simulink model "s32k344_mcb_sensorless_s32ct"  (R2024b)
settings: Solver=FixedStepAuto  StartTime=0.0  StopTime=20  RelTol=1e-3  EnableMultiTasking=on
PreLoadFcn:
  | % NXP_MBDT_S32K3 callback: DO NOT REMOVE
  | mbd_s32k3.common.nxp.model_callbacks.preLoadFcn();
  | 
  | s32k344Data;
  | mcbSensorlessData;
PostLoadFcn:
  | % NXP_MBDT_S32K3 callback: DO NOT REMOVE
  | mbd_s32k3.common.nxp.model_callbacks.postLoadFcn();
InitFcn:
  | % NXP_MBDT_S32K3 callback: DO NOT REMOVE
  | mbd_s32k3.common.nxp.model_callbacks.initFcn();
values from neighbouring files (symbols this model uses):
  PWM_DutyScale = 32768    [s32k344Data.m]
  PWM_Period = 8000    [s32k344Data.m]
  Ts_motor = T_pwm    (= 5e-05)    [s32k344Data.m]
  Ts_SerialIn = 0.1    [s32k344Data.m]
  Ts_SerialOut = 0.01    [s32k344Data.m]
  Ts_SysControl = 0.1    [mcbSensorlessData.m]
undefined symbols (not defined in the file or in its folder): inverter, LogicOutputId, pmsm, Value
libraries: mbd_s32k3_io_library x14, mbd_s32k3_cdd_library x4, simulink x4, mbd_s32k3_isr_library x1, mbd_s32k3_utility_library x1
(part 3 of 3)

== system s32k344_mcb_sensorless_s32ct/Control/HW INT/CodeGeneration/ADC_INT/ADC_IRQHandler/Fault Detection ==
  VDC : Inport
  Constant : Constant  Value=pmsm.V_max/inverter.MaxADCCnt  OutDataTypeStr=single  SampleTime=-1
  Data Type Conversion : DataTypeConversion  OutDataTypeStr=single  SaturateOnIntegerOverflow=off  RndMeth=Floor
  FAILURE : Subsystem  TreatAsAtomicUnit=on
  If : If  IfExpression=(u1 < underVoltage) | (u1 > overVoltage)  ShowElse=off
  Product : Product  OutDataTypeStr=single
  wires:
  VDC/1 -> Data Type Conversion/1
  Data Type Conversion/1 -> Product/1
  Constant/1 -> Product/2
  Product/1 -> If/1  "Vdc"
  If/1 -> FAILURE/Action

== system s32k344_mcb_sensorless_s32ct/Control/HW INT/CodeGeneration/ADC_INT/ADC_IRQHandler/Fault Detection/FAILURE ==
  Action Port : ActionPort  ActionPortLabel=if((u1 < underVoltage) | (u1 > overVoltage))
  Data Store Read : DataStoreRead  DataStoreName=FAULT  IndexOptions=Index vector (dialog)  Indices=1  OutputSizes=1
  If : If  IfExpression=u1 == 0  ShowElse=off
  If Action Subsystem : Subsystem  TreatAsAtomicUnit=on
  wires:
  Data Store Read/1 -> If/1
  If/1 -> If Action Subsystem/Action

== system s32k344_mcb_sensorless_s32ct/Control/HW INT/CodeGeneration/ADC_INT/ADC_IRQHandler/Fault Detection/FAILURE/If Action Subsystem ==
  Action Port : ActionPort  ActionPortLabel=if(u1 == 0)
  Data Store Write : DataStoreWrite  DataStoreName=FAULT  IndexOptions=Index vector (dialog)  Indices=1  OutputSizes=1
  Disable LCU : Subsystem  Priority=3
  NOT_OK : Constant  OutDataTypeStr=boolean
  wires:
  NOT_OK/1 -> Data Store Write/1

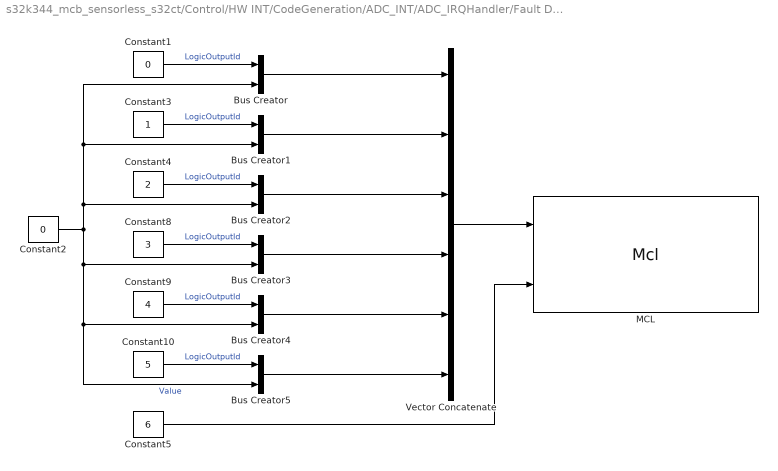
== system s32k344_mcb_sensorless_s32ct/Control/HW INT/CodeGeneration/ADC_INT/ADC_IRQHandler/Fault Detection/FAILURE/If Action Subsystem/Disable LCU ==
  Bus Creator{,1..5} (6 alike) : BusCreator  Inputs=LogicOutputId,Value  OutDataTypeStr=Bus: Mcl_LcuSyncOutputValueType  NonVirtualBus=on
  Constant1 : Constant  Value=0  OutDataTypeStr=uint8
  Constant10 : Constant  Value=5  OutDataTypeStr=uint8
  Constant2 : Constant  Value=0  OutDataTypeStr=uint16
  Constant3 : Constant  OutDataTypeStr=uint8
  Constant4 : Constant  Value=2  OutDataTypeStr=uint8
  Constant5 : Constant  Value=6  OutDataTypeStr=uint8
  Constant8 : Constant  Value=3  OutDataTypeStr=uint8
  Constant9 : Constant  Value=4  OutDataTypeStr=uint8
  MCL : mbd_s32k3_cdd_library/Mcl  Priority=2  api_func=Mcl_SetLcuSyncOutputEnable  logicInput=LCU_LOGIC_INPUT_0  logicOutput=LCU_LOGIC_OUTPUT_0  logicInstance=LCU_LOGIC_INSTANCE_0  emiosInstance=EMIOS_0  ftmInstance=FTM0  logicChannel=EMIOS_0_EmiosMclMasterBus_0  prescalerType=MCL_EMIOS_PRESCALER  dmaLogicInstance=No DMA logic instances configured  dmaLogicChannel=DMA_LOGIC_CH_0  dmaInstanceCommandType=MCL_DMA_INST_STOP  dmaChannelCommandType=MCL_DMA_CH_START_REQUEST  dmaScatterGatherElement=No DMA Scatter Gather elements configured  dmaChannelInfo=MCL_DMA_CH_GET_SOURCE_ADDRESS  text=<binary blob, 55810 chars, not shown>
      settings: SourceProductName=CDD Blocks
  Vector Concatenate : Concatenate  NumInputs=6
  wires:
  Constant4/1 -> Bus Creator2/1  "LogicOutputId"
  Constant2/1 -> Bus Creator/2, Bus Creator1/2, Bus Creator2/2, Bus Creator5/2, Bus Creator4/2, Bus Creator3/2  "Value"
  Constant1/1 -> Bus Creator/1  "LogicOutputId"
  Bus Creator4/1 -> Vector Concatenate/5
  Constant9/1 -> Bus Creator4/1  "LogicOutputId"
  Bus Creator/1 -> Vector Concatenate/1
  Constant5/1 -> MCL/2
  Constant8/1 -> Bus Creator3/1  "LogicOutputId"
  Bus Creator2/1 -> Vector Concatenate/3
  Constant10/1 -> Bus Creator5/1  "LogicOutputId"
  Bus Creator5/1 -> Vector Concatenate/6
  Vector Concatenate/1 -> MCL/1
  Constant3/1 -> Bus Creator1/1  "LogicOutputId"
  Bus Creator1/1 -> Vector Concatenate/2
  Bus Creator3/1 -> Vector Concatenate/4
